simulink model "walkgen"  (Simulink 7.0)
settings: Solver=FixedStepDiscrete  StartTime=0.0  StopTime=10  FixedStep=1e-3  RelTol=1e-3
Description:
  | Bringing in C++ Code into a C++ S-function Including Code Generation Support
CloseFcn:
  | rtwprivate ssgencode ModelCloseRequest walkgen
settings Model: Creator=The MathWorks Inc.  LastModifiedBy=herd_an  ExtModeTrigMode=oneshot  ExtModeArmWhenConnect=off  ExtModeAutoUpdateStatusClock=off
settings DataIOCC: LimitDataPoints=off  SaveOutput=off  SignalLogging=off  SaveTime=off  SignalLoggingName=logsOut
settings OptimizationCC: EnforceIntegerDowncast=off  StateBitsets=on  DataBitsets=on  UseTempVars=on  BufferReusableBoundary=off
settings DebuggingCC: SaveWithParameterizedLinksMsg=none  SignalResolutionControl=TryResolveAllWithWarning  SolverPrmCheckMsg=none  MultiTaskDSMMsg=warning  MultiTaskCondExecSysMsg=none  SigSpecEnsureSampleTimeMsg=none  StrictBusMsg=None
settings HardwareCC: ProdHWDeviceType=Specified  TargetHWDeviceType=32-bit Generic  ProdEqTarget=off
settings RTWCC: GenerateReport=on  RTWVerbose=off  ProcessScript=grt_make_rtw_hook  CustomSourceCode="#include \"sfun_cppcount_cpp.h\""  CustomInclude=../../../../simulink/src  CustomSource=sfun_cppcount_cpp.cpp  LaunchReport=on  TargetLang=C++  IncludeERTFirstTime=on
settings CodeAppCC: ForceParamTrailComments=on  CustomSymbolStrFcn=$F$N$M
settings GRTTargetCC: TargetFcnLib=ansi_tfl_tmw.mat

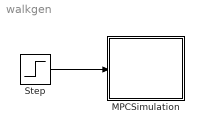
== system walkgen ==
  MPCSimulation : Subsystem  Orientation=up
  Step : Step  Time=3  SampleTime=0.005
  wires:
  Step/1 -> MPCSimulation/Enable

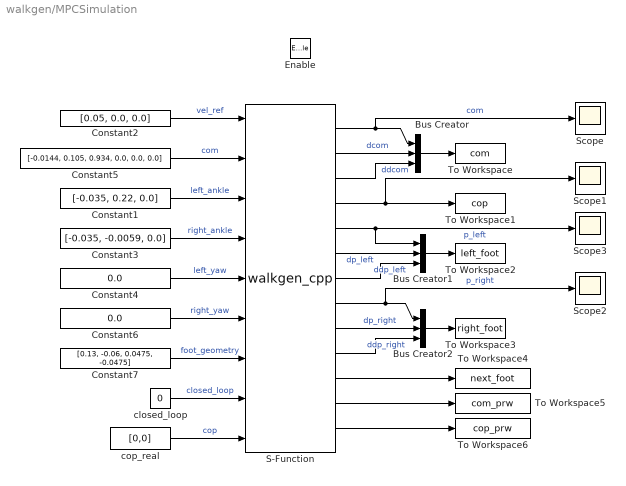
== system walkgen/MPCSimulation ==
  Enable : EnablePort
  Bus Creator : BusCreator  Inputs=3
  Bus Creator1 : BusCreator  Inputs=3
  Bus Creator2 : BusCreator  Inputs=3
  Constant1 : Constant  Value=[-0.035, 0.22, 0.0]  OutDataType=sfix(16)  OutScaling=2^0
  Constant2 : Constant  Value=[0.05, 0.0, 0.0]  OutDataType=sfix(16)  OutScaling=2^0
  Constant3 : Constant  Value=[-0.035, -0.0059, 0.0]  OutDataType=sfix(16)  OutScaling=2^0
  Constant4 : Constant  Value=0.0  OutDataType=sfix(16)  OutScaling=2^0
  Constant5 : Constant  Value=[-0.0144, 0.105, 0.934, 0.0, 0.0, 0.0]  OutDataType=sfix(16)  OutScaling=2^0
  Constant6 : Constant  Value=0.0  OutDataType=sfix(16)  OutScaling=2^0
  Constant7 : Constant  Value=[0.13, -0.06, 0.0475, -0.0475]  OutDataType=sfix(16)  OutScaling=2^0
  S-Function : S-Function  FunctionName=walkgen_cpp
  Scope{,1..3} (4 alike) : Scope
      Scope settings: TimeRange=0.007766893178016154  YMin=0.05  YMax=0.95
      Scope2 settings: SaveName=ScopeData2
      Scope3 settings: SaveName=ScopeData3
  To Workspace : ToWorkspace  VariableName=com  SampleTime=-1  SaveFormat=Structure With Time
  To Workspace1 : ToWorkspace  VariableName=cop  SampleTime=-1  SaveFormat=Structure With Time
  To Workspace2 : ToWorkspace  VariableName=left_foot  SampleTime=-1  SaveFormat=Structure With Time
  To Workspace3 : ToWorkspace  VariableName=right_foot  SampleTime=-1  SaveFormat=Structure With Time
  To Workspace4 : ToWorkspace  VariableName=next_foot  SampleTime=-1  SaveFormat=Structure With Time
  To Workspace5 : ToWorkspace  VariableName=com_prw  SampleTime=-1  SaveFormat=Structure With Time
  To Workspace6 : ToWorkspace  VariableName=cop_prw  SampleTime=-1  SaveFormat=Structure With Time
  closed_loop : Constant  Value=0  OutDataType=sfix(16)  OutScaling=2^0
  cop_real : Constant  Value=[0,0]  OutDataType=sfix(16)  OutScaling=2^0
  wires:
  S-Function/1 -> Bus Creator/1, Scope/1  "com"
  S-Function/4 -> To Workspace1/1, Scope1/1
  Bus Creator2/1 -> To Workspace3/1
  S-Function/9 -> Bus Creator2/2  "dp_right"
  Bus Creator/1 -> To Workspace/1
  S-Function/2 -> Bus Creator/2  "dcom"
  S-Function/3 -> Bus Creator/3  "ddcom"
  Bus Creator1/1 -> To Workspace2/1
  Constant2/1 -> S-Function/1  "vel_ref"
  Constant5/1 -> S-Function/2  "com"
  Constant1/1 -> S-Function/3  "left_ankle"
  Constant3/1 -> S-Function/4  "right_ankle"
  Constant4/1 -> S-Function/5  "left_yaw"
  Constant6/1 -> S-Function/6  "right_yaw"
  Constant7/1 -> S-Function/7  "foot_geometry"
  S-Function/11 -> To Workspace4/1
  S-Function/10 -> Bus Creator2/3  "ddp_right"
  S-Function/8 -> Bus Creator2/1, Scope2/1  "p_right"
  S-Function/5 -> Scope3/1, Bus Creator1/1  "p_left"
  S-Function/6 -> Bus Creator1/2  "dp_left"
  S-Function/7 -> Bus Creator1/3  "ddp_left"
  S-Function/12 -> To Workspace5/1
  closed_loop/1 -> S-Function/8  "closed_loop"
  cop_real/1 -> S-Function/9  "cop"
  S-Function/13 -> To Workspace6/1
